simulink model "base_simulink"  (R2014b)
settings: Solver=ode45  StartTime=0.0  StopTime=0.1  RelTol=1e-3
values from neighbouring files (symbols this model uses):
  Bm = 0.0    (= 0)    [base.m]    (also in base_parameter.m; lqr_parameter.m; pid_perameter.m)
  Jm = 24.5*10^-7    (= 2.45e-06)    [base.m]    (also in base_parameter.m = 1.08e-06; lqr_parameter.m = 1.08e-06; pid_perameter.m)
  Ke = 173*0.10472    (= 18.11656)    [base.m]    (also in base_parameter.m = 0.0234050839587; lqr_parameter.m = 0.0234050839587; pid_perameter.m = 173)
  Kt = 55.2*10^-3    (= 0.0552)    [base.m]    (also in base_parameter.m = 0.00285; lqr_parameter.m = 0.00285; pid_perameter.m)
  La = 5.02*10^-3    (= 0.00502)    [base.m]    (also in base_parameter.m = 0.000238; lqr_parameter.m = 0.000238; pid_perameter.m)
  Ra = 40    [base.m]    (also in base_parameter.m = 2.32; lqr_parameter.m = 2.32; pid_perameter.m)
settings Model: Creator=Admin  LastModifiedBy=Admin

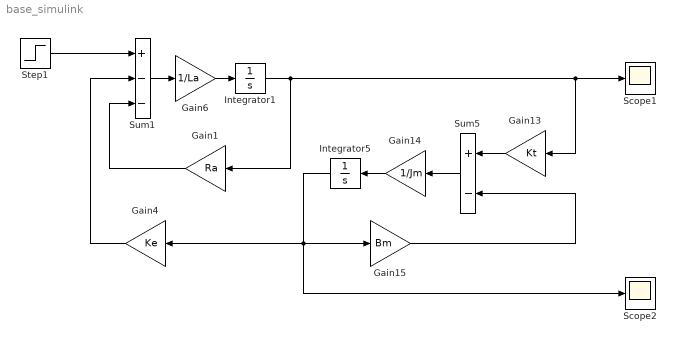
== system base_simulink ==
  Gain1 : Gain  Gain=Ra
  Gain13 : Gain  Gain=Kt
  Gain14 : Gain  Gain=1/Jm
  Gain15 : Gain  Gain=Bm
  Gain4 : Gain  Gain=Ke
  Gain6 : Gain  Gain=1/La
  Integrator1 : Integrator
  Integrator5 : Integrator
  Scope1 : Scope
      settings: YMin=0  YMax=10
  Scope2 : Scope
      settings: YMin=0  YMax=10
  Step1 : Step  Time=0  After=24  SampleTime=0
  Sum1 : Sum  Inputs=+--
  Sum5 : Sum  Inputs=+-
  wires:
  Gain4/1 -> Sum1/2
  Sum1/1 -> Gain6/1
  Gain6/1 -> Integrator1/1
  Gain1/1 -> Sum1/3
  Gain13/1 -> Sum5/1
  Sum5/1 -> Gain14/1
  Gain14/1 -> Integrator5/1
  Gain15/1 -> Sum5/2
  Integrator1/1 -> Scope1/1, Gain13/1, Gain1/1
  Integrator5/1 -> Scope2/1, Gain15/1, Gain4/1
  Step1/1 -> Sum1/1
